simulink model "requirements"  (R2022a)
settings: Solver=FixedStepAuto  StartTime=0.0  StopTime=10.0  FixedStep=1e-3  RelTol=1e-3  EnableMultiTasking=on
settings Model: ExtModeTrigDuration=5  Creator=zaree  LastModifiedBy=zaree
settings OptimizationCC: EnhancedBackFolding=on  PassReuseOutputArgsAs=Individual arguments  ZeroExternalMemoryAtStartup=off  ZeroInternalMemoryAtStartup=off  MaxStackSize=64  OptimizeBlockOrder=speed  DifferentSizesBufferReuse=on  OptimizationCustomize=off  EfficientTunableParamExpr=on
settings DebuggingCC: ParameterTunabilityLossMsg=error
settings HardwareCC: ProdBitPerPointer=32  ProdBitPerSizeT=32  ProdBitPerPtrDiffT=32  ProdLargestAtomicInteger=Long  ProdLargestAtomicFloat=Double  ProdWordSize=32  ProdHWDeviceType=ARM Compatible->ARM Cortex
settings SFSimCC: MATLABDynamicMemAlloc=off
settings RTWCC: SystemTargetFile=ert.tlc  HardwareBoard=NXP FRDM-K64F  TLCOptions="-aInlineSetEventsForThisBaseRateFcn=TLC_FALSE -aSuppressMultiTaskScheduler=TLC_FALSE  -aRateBasedStepFcn=0"  TemplateMakefile=ert_default_tmf  Toolchain=GNU Tools for ARM Embedded Processors
settings CodeAppCC: ForceParamTrailComments=on  IgnoreCustomStorageClasses=off  OperatorAnnotations=on  SimulinkDataObjDesc=on  SFDataObjDesc=on  InsertBlockDesc=on
settings ERTTargetCC: ExtModeTransport=4  ExtModeMexFile=sendToCommService

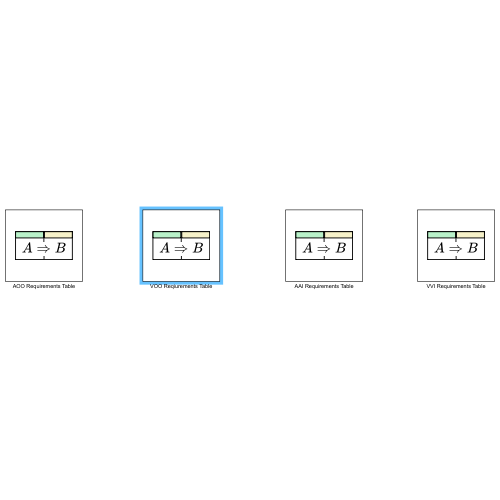
[thumbnail: Simulink's stored preview of the top-level diagram]
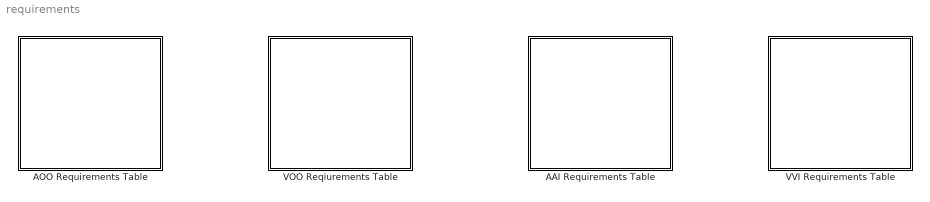
== system requirements ==
  AAI Requirements Table : Requirements Table  TreatAsAtomicUnit=on
  AOO Requirements Table : Requirements Table  TreatAsAtomicUnit=on
  VOO Reqiurements Table : Requirements Table  TreatAsAtomicUnit=on
  VVI Requirements Table : Requirements Table  TreatAsAtomicUnit=on

== stateflow chart requirements/VOO Reqiurements Table ==
  (default) -> (junction 1073741860)
  (junction 1073741860) -> (junction 1073741861) : {
      | % SF_REQ_REV_07
      | }
  (junction 1073741861) -> (junction 1073741863) : {
      | % HEADER_ASSIGNMENTS
      |
      | }
  (junction 1073741863) -> (junction 1073741865) : {
      | % START_A_4
      | }
  (junction 1073741865) -> (junction 1073741867) : {
      | }
  (junction 1073741867) -> (junction 1073741869)
  (junction 1073741869) -> (junction 1073741871) : {
      | }
  (junction 1073741871) -> (junction 1073741873) : {
      | % END_A_4
      | }
  (junction 1073741873) -> (junction 1073741898) : {
      | % START_R_1
      | }
  (junction 1073741898) -> (junction 1073741900) : {
      | }
  (junction 1073741900) -> (junction 1073741902) : {
      |
      |
      | }
  (junction 1073741902) -> (junction 1073741904) : {
      | }
  (junction 1073741904) -> (junction 1073741906) : {
      | % END_R_1
      | }
  (junction 1073741906) -> (junction 1073741910) : {
      | % START_R_7
      | }
  (junction 1073741910) -> (junction 1073741912) : {
      | }
  (junction 1073741912) -> (junction 1073741914) : {
      |
      |
      | }
  (junction 1073741914) -> (junction 1073741916) : {
      | }
  (junction 1073741916) -> (junction 1073741918) : {
      | % END_R_7
      | }

== stateflow chart requirements/VVI Requirements Table ==
  (default) -> (junction 1073741999)
  (junction 1073741999) -> (junction 1073742000) : {
      | % SF_REQ_REV_07
      | }
  (junction 1073742000) -> (junction 1073742002) : {
      | % HEADER_ASSIGNMENTS
      |
      | }
  (junction 1073742002) -> (junction 1073742004) : {
      | % START_A_4
      | }
  (junction 1073742004) -> (junction 1073742006) : {
      | }
  (junction 1073742006) -> (junction 1073742008)
  (junction 1073742008) -> (junction 1073742010) : {
      | }
  (junction 1073742010) -> (junction 1073742030) : {
      | % END_A_4
      | }
  (junction 1073742030) -> (junction 1073742066) : {
      | % START_R_10
      | }
  (junction 1073742066) -> (junction 1073742068) : {
      | }
  (junction 1073742068) -> (junction 1073742070) : {
      |
      |
      | }
  (junction 1073742070) -> (junction 1073742072) : {
      | }
  (junction 1073742072) -> (junction 1073742074) : {
      | % END_R_10
      | }
  (junction 1073742074) -> (junction 1073742078) : {
      | % START_R_1
      | }
  (junction 1073742078) -> (junction 1073742080) : {
      | }
  (junction 1073742080) -> (junction 1073742082)
  (junction 1073742082) -> (junction 1073742084) [order 1] : [duration((PACE_CHARGE_CTRL == 1) && (VENT_PACE_CTRL == 1) && (VENT_GND_CTRL == 0) && (PACE_GND_CTRL == 0 ) && (Z_VENT_CTRL == 0) && (VENT_CMP_DETECT ==1)) >= f_waitInterval]
  (junction 1073742082) -> (junction 1073742090) [order 2]
  (junction 1073742084) -> (junction 1073742086) : {
      | reqtable_postcondition((PACE_CHARGE_CTRL == 1) && (VENT_PACE_CTRL == 1) && (VENT_GND_CTRL == 0) && (PACE_GND_CTRL == 0) && (Z_VENT_CTRL == 0) && (VENT_CMP_DETECT ==1), 'R:2');
      | SENSE
      |
      | }
  (junction 1073742086) -> (junction 1073742088) : {
      | }
  (junction 1073742088) -> (junction 1073742090)
  (junction 1073742090) -> (junction 1073742092)
  (junction 1073742092) -> (junction 1073742094) : {
      | % END_R_1
      | }
  (junction 1073742094) -> (junction 1073742045) : {
      | % START_R_7
      | }
  (junction 1073742045) -> (junction 1073742047) : {
      | }
  (junction 1073742047) -> (junction 1073742049)
  (junction 1073742049) -> (junction 1073742051) [order 1] : [duration((PACE_CHARGE_CTRL == 1) && (VENT_PACE_CTRL == 1) && (VENT_GND_CTRL == 0) && (PACE_GND_CTRL == 0) && (Z_VENT_CTRL == 0) && (VENT_CMP_DETECT ==0)) >= f_waitInterval]
  (junction 1073742049) -> (junction 1073742057) [order 2]
  (junction 1073742051) -> (junction 1073742053) : {
      | reqtable_postcondition((PACE_CHARGE_CTRL == 0) && (VENT_PACE_CTRL == 1) && (VENT_GND_CTRL == 0) && (PACE_GND_CTRL == 1) && (Z_VENT_CTRL == 0) && (VENT_CMP_DETECT ==1), 'R:3');
      | PACE
      |
      | }
  (junction 1073742053) -> (junction 1073742055) : {
      | }
  (junction 1073742055) -> (junction 1073742057)
  (junction 1073742057) -> (junction 1073742059)
  (junction 1073742059) -> (junction 1073742061) : {
      | % END_R_7
      | }

== stateflow chart requirements/AOO Requirements Table ==
  (default) -> (junction 1073742591)
  (junction 1073742591) -> (junction 1073742592) : {
      | % SF_REQ_REV_07
      | }
  (junction 1073742592) -> (junction 1073742594) : {
      | % HEADER_ASSIGNMENTS
      |
      | }
  (junction 1073742594) -> (junction 1073742596) : {
      | % START_A_4
      | }
  (junction 1073742596) -> (junction 1073742598) : {
      | }
  (junction 1073742598) -> (junction 1073742600)
  (junction 1073742600) -> (junction 1073742602) : {
      | }
  (junction 1073742602) -> (junction 1073742604) : {
      | % END_A_4
      | }
  (junction 1073742604) -> (junction 1073742606) : {
      | % START_R_1
      | }
  (junction 1073742606) -> (junction 1073742608) : {
      | }
  (junction 1073742608) -> (junction 1073742610)
  (junction 1073742610) -> (junction 1073742612) [order 1] : [(PACE_CHARGE_CTRL == 0) && (ATR_CHARGE_CTRL == 1) && (ATR_GND_CTRL == 0) && (PACE_GND_CTRL == 1) && (Z_ATR_CTRL == 0)]
  (junction 1073742610) -> (junction 1073742618) [order 2]
  (junction 1073742612) -> (junction 1073742614) : {
      | reqtable_postcondition((PACE_CHARGE_CTRL == 1) && (ATR_PACE_CTRL == 0) && (ATR_GND_CTRL == 1) && (PACE_GND_CTRL == 1) && (Z_ATR_CTRL == 0), 'R:1');
      |
      |
      | }
  (junction 1073742614) -> (junction 1073742616) : {
      | }
  (junction 1073742616) -> (junction 1073742618)
  (junction 1073742618) -> (junction 1073742620)
  (junction 1073742620) -> (junction 1073742622) : {
      | % END_R_1
      | }
  (junction 1073742622) -> (junction 1073742624) : {
      | % START_R_7
      | }
  (junction 1073742624) -> (junction 1073742626) : {
      | }
  (junction 1073742626) -> (junction 1073742628)
  (junction 1073742628) -> (junction 1073742630) [order 1] : [(PACE_CHARGE_CTRL == 1) && (ATR_PACE_CTRL==0) && (ATR_GND_CTRL==1) && (PACE_GND_CTRL == 1) && (Z_ATR_CTRL == 0)]
  (junction 1073742628) -> (junction 1073742636) [order 2]
  (junction 1073742630) -> (junction 1073742632) : {
      | reqtable_postcondition((PACE_CHARGE_CTRL == 0) && (ATR_CHARGE_CTRL == 1) && (ATR_GND_CTRL == 0) && (PACE_GND_CTRL == 1) && (Z_ATR_CTRL == 0), 'R:2');
      |
      |
      | }
  (junction 1073742632) -> (junction 1073742634) : {
      | }
  (junction 1073742634) -> (junction 1073742636)
  (junction 1073742636) -> (junction 1073742638)
  (junction 1073742638) -> (junction 1073742640) : {
      | % END_R_7
      | }
  (junction 1073742640) -> (junction 1073742642) : {
      | % START_R_10
      | }
  (junction 1073742642) -> (junction 1073742644) : {
      | }
  (junction 1073742644) -> (junction 1073742646)
  (junction 1073742646) -> (junction 1073742648) [order 1] : [(PACE_CHARGE_CTRL == 0) && (VENT_PACE_CTRL == 1) && (VENT_GND_CTRL == 0) && (PACE_GND_CTRL == 1) && (Z_VENT_CTRL == 0)]
  (junction 1073742646) -> (junction 1073742654) [order 2]
  (junction 1073742648) -> (junction 1073742650) : {
      | reqtable_postcondition((PACE_CHARGE_CTRL == 1) && (VENT_CHARGE_CTRL == 0) && (VENT_GND_CTRL == 1) && (PACE_GND_CTRL == 1) && (Z_VENT_CTRL == 0), 'R:3');
      |
      |
      | }
  (junction 1073742650) -> (junction 1073742652) : {
      | }
  (junction 1073742652) -> (junction 1073742654)
  (junction 1073742654) -> (junction 1073742656)
  (junction 1073742656) -> (junction 1073742658) : {
      | % END_R_10
      | }
  (junction 1073742658) -> (junction 1073742660) : {
      | % START_R_13
      | }
  (junction 1073742660) -> (junction 1073742662) : {
      | }
  (junction 1073742662) -> (junction 1073742664)
  (junction 1073742664) -> (junction 1073742666) [order 1] : [(PACE_CHARGE_CTRL == 1) && (VENT_PACE_CTRL == 0) && (VENT_GND_CTRL == 1) && (PACE_GND_CTRL == 1) && (Z_VENT_CTRL == 0)]
  (junction 1073742664) -> (junction 1073742672) [order 2]
  (junction 1073742666) -> (junction 1073742668) : {
      | reqtable_postcondition((PACE_CHARGE_CTRL == 0) && (VENT_CHARGE_CTRL == 1) && (VENT_GND_CTRL == 0) && (PACE_GND_CTRL == 1) && (Z_VENT_CTRL == 0), 'R:4');
      |
      |
      | }
  (junction 1073742668) -> (junction 1073742670) : {
      | }
  (junction 1073742670) -> (junction 1073742672)
  (junction 1073742672) -> (junction 1073742674)
  (junction 1073742674) -> (junction 1073742676) : {
      | % END_R_13
      | }
  (junction 1073742676) -> (junction 1073742766) : {
      | % START_R_22
      | }
  (junction 1073742766) -> (junction 1073742768) : {
      | }
  (junction 1073742768) -> (junction 1073742770)
  (junction 1073742770) -> (junction 1073742772) [order 1] : [duration((PACE_CHARGE_CTRL == 1) && (ATR_PACE_CTRL == 1) && (ATR_GND_CTRL == 0) && (PACE_GND_CTRL == 0 ) && (Z_ATR_CTRL == 0) && (ATR_CMP_DETECT ==1)) >= VRP]
  (junction 1073742770) -> (junction 1073742778) [order 2]
  (junction 1073742772) -> (junction 1073742774) : {
      | reqtable_postcondition((PACE_CHARGE_CTRL == 1) && (ATR_PACE_CTRL == 1) && (ATR_GND_CTRL == 0) && (PACE_GND_CTRL == 0) && (Z_ATR_CTRL == 0) && (ATR_CMP_DETECT ==1), 'R:5');
      | SENSE
      |
      | }
  (junction 1073742774) -> (junction 1073742776) : {
      | }
  (junction 1073742776) -> (junction 1073742778)
  (junction 1073742778) -> (junction 1073742780)
  (junction 1073742780) -> (junction 1073742782) : {
      | % END_R_22
      | }
  (junction 1073742782) -> (junction 1073742787) : {
      | % START_R_25
      | }
  (junction 1073742787) -> (junction 1073742789) : {
      | }
  (junction 1073742789) -> (junction 1073742791)
  (junction 1073742791) -> (junction 1073742793) [order 1] : [duration((PACE_CHARGE_CTRL == 1) && (ATR_PACE_CTRL == 1) && (ATR_GND_CTRL == 0) && (PACE_GND_CTRL == 0) && (Z_ATR_CTRL == 0) && (ATR_CMP_DETECT ==0)) >= NOT_Atrium_Pulse_Width - VRP]
  (junction 1073742791) -> (junction 1073742799) [order 2]
  (junction 1073742793) -> (junction 1073742795) : {
      | reqtable_postcondition((PACE_CHARGE_CTRL == 0) && (ATR_PACE_CTRL == 1) && (ATR_GND_CTRL == 0) && (PACE_GND_CTRL == 1) && (Z_ATR_CTRL == 0) && (ATR_CMP_DETECT ==0), 'R:6');
      | PACE
      |
      | }
  (junction 1073742795) -> (junction 1073742797) : {
      | }
  (junction 1073742797) -> (junction 1073742799)
  (junction 1073742799) -> (junction 1073742801)
  (junction 1073742801) -> (junction 1073742803) : {
      | % END_R_25
      | }
  (junction 1073742803) -> (junction 1073742820) : {
      | % START_R_34
      | }
  (junction 1073742820) -> (junction 1073742822) : {
      | }
  (junction 1073742822) -> (junction 1073742824)
  (junction 1073742824) -> (junction 1073742826) [order 1] : [duration((PACE_CHARGE_CTRL == 0) && (ATR_PACE_CTRL == 1) && (ATR_GND_CTRL == 0) && (PACE_GND_CTRL == 1) && (Z_ATR_CTRL == 0) && (ATR_CMP_DETECT ==1)) >= Atrium_Pulse_Width]
  (junction 1073742824) -> (junction 1073742832) [order 2]
  (junction 1073742826) -> (junction 1073742828) : {
      | reqtable_postcondition((PACE_CHARGE_CTRL == 1) && (ATR_PACE_CTRL == 1) && (ATR_GND_CTRL == 0) && (PACE_GND_CTRL == 0 ) && (Z_ATR_CTRL == 0) && (ATR_CMP_DETECT ==1), 'R:7');
      | SENSE
      |
      | }
  (junction 1073742828) -> (junction 1073742830) : {
      | }
  (junction 1073742830) -> (junction 1073742832)
  (junction 1073742832) -> (junction 1073742834)
  (junction 1073742834) -> (junction 1073742836) : {
      | % END_R_34
      | }
  (junction 1073742836) -> (junction 1073742724) : {
      | % START_R_28
      | }
  (junction 1073742724) -> (junction 1073742726) : {
      | }
  (junction 1073742726) -> (junction 1073742728)
  (junction 1073742728) -> (junction 1073742730) [order 1] : [duration((PACE_CHARGE_CTRL == 1) && (VENT_PACE_CTRL == 1) && (VENT_GND_CTRL == 0) && (PACE_GND_CTRL == 0 ) && (Z_VENT_CTRL == 0) && (VENT_CMP_DETECT ==1)) >= VRP]
  (junction 1073742728) -> (junction 1073742736) [order 2]
  (junction 1073742730) -> (junction 1073742732) : {
      | reqtable_postcondition((PACE_CHARGE_CTRL == 1) && (VENT_PACE_CTRL == 1) && (VENT_GND_CTRL == 0) && (PACE_GND_CTRL == 0) && (Z_VENT_CTRL == 0) && (VENT_CMP_DETECT ==1), 'R:8');
      | SENSE
      |
      | }
  (junction 1073742732) -> (junction 1073742734) : {
      | }
  (junction 1073742734) -> (junction 1073742736)
  (junction 1073742736) -> (junction 1073742738)
  (junction 1073742738) -> (junction 1073742740) : {
      | % END_R_28
      | }
  (junction 1073742740) -> (junction 1073742745) : {
      | % START_R_31
      | }
  (junction 1073742745) -> (junction 1073742747) : {
      | }
  (junction 1073742747) -> (junction 1073742749)
  (junction 1073742749) -> (junction 1073742751) [order 1] : [duration((PACE_CHARGE_CTRL == 1) && (VENT_PACE_CTRL == 1) && (VENT_GND_CTRL == 0) && (PACE_GND_CTRL == 0) && (Z_VENT_CTRL == 0) && (VENT_CMP_DETECT ==0)) >= NOT_Ventricular_Pulse_Width - VRP]
  (junction 1073742749) -> (junction 1073742757) [order 2]
  (junction 1073742751) -> (junction 1073742753) : {
      | reqtable_postcondition((PACE_CHARGE_CTRL == 0) && (VENT_PACE_CTRL == 1) && (VENT_GND_CTRL == 0) && (PACE_GND_CTRL == 1) && (Z_VENT_CTRL == 0) && (VENT_CMP_DETECT ==0), 'R:9');
      | PACE
      |
      | }
  (junction 1073742753) -> (junction 1073742755) : {
      | }
  (junction 1073742755) -> (junction 1073742757)
  (junction 1073742757) -> (junction 1073742759)
  (junction 1073742759) -> (junction 1073742761) : {
      | % END_R_31
      | }
  (junction 1073742761) -> (junction 1073742853) : {
      | % START_R_37
      | }
  (junction 1073742853) -> (junction 1073742855) : {
      | }
  (junction 1073742855) -> (junction 1073742857)
  (junction 1073742857) -> (junction 1073742859) [order 1] : [duration((PACE_CHARGE_CTRL == 0) && (VENT_PACE_CTRL == 1) && (VENT_GND_CTRL == 0) && (PACE_GND_CTRL == 1) && (Z_VENT_CTRL == 0) && (VENT_CMP_DETECT ==0)) >= Ventricular_Pulse_Width]
  (junction 1073742857) -> (junction 1073742865) [order 2]
  (junction 1073742859) -> (junction 1073742861) : {
      | reqtable_postcondition((PACE_CHARGE_CTRL == 1) && (VENT_PACE_CTRL == 1) && (VENT_GND_CTRL == 0) && (PACE_GND_CTRL == 0 ) && (Z_VENT_CTRL == 0) && (VENT_CMP_DETECT ==1), 'R:10');
      | SENSE
      |
      | }
  (junction 1073742861) -> (junction 1073742863) : {
      | }
  (junction 1073742863) -> (junction 1073742865)
  (junction 1073742865) -> (junction 1073742867)
  (junction 1073742867) -> (junction 1073742869) : {
      | % END_R_37
      | }

== stateflow chart requirements/AAI Requirements Table ==
  (default) -> (junction 1073741963)
  (junction 1073741963) -> (junction 1073741964) : {
      | % SF_REQ_REV_07
      | }
  (junction 1073741964) -> (junction 1073741966) : {
      | % HEADER_ASSIGNMENTS
      |
      | }
  (junction 1073741966) -> (junction 1073741968) : {
      | % START_A_4
      | }
  (junction 1073741968) -> (junction 1073741970) : {
      | }
  (junction 1073741970) -> (junction 1073741972)
  (junction 1073741972) -> (junction 1073741974) : {
      | }
  (junction 1073741974) -> (junction 1073741976) : {
      | % END_A_4
      | }
  (junction 1073741976) -> (junction 1073741978) : {
      | % START_R_1
      | }
  (junction 1073741978) -> (junction 1073741980) : {
      | }
  (junction 1073741980) -> (junction 1073741982)
  (junction 1073741982) -> (junction 1073741984) [order 1] : [duration((PACE_CHARGE_CTRL == 1) && (ATR_PACE_CTRL == 1) && (ATR_GND_CTRL == 0) && (PACE_GND_CTRL == 0 ) && (Z_ATR_CTRL == 0) && (ATR_CMP_DETECT ==1)) >= f_waitInterval]
  (junction 1073741982) -> (junction 1073741990) [order 2]
  (junction 1073741984) -> (junction 1073741986) : {
      | reqtable_postcondition((PACE_CHARGE_CTRL == 1) && (ATR_PACE_CTRL == 1) && (ATR_GND_CTRL == 0) && (PACE_GND_CTRL == 0) && (Z_ATR_CTRL == 0) && (ATR_CMP_DETECT ==1), 'R:1');
      | SENSE
      |
      | }
  (junction 1073741986) -> (junction 1073741988) : {
      | }
  (junction 1073741988) -> (junction 1073741990)
  (junction 1073741990) -> (junction 1073741992)
  (junction 1073741992) -> (junction 1073741994) : {
      | % END_R_1
      | }
  (junction 1073741994) -> (junction 1073741996) : {
      | % START_R_7
      | }
  (junction 1073741996) -> (junction 1073741998) : {
      | }
  (junction 1073741998) -> (junction 1073742000)
  (junction 1073742000) -> (junction 1073742002) [order 1] : [duration((PACE_CHARGE_CTRL == 1) && (ATR_PACE_CTRL == 1) && (ATR_GND_CTRL == 0) && (PACE_GND_CTRL == 0) && (Z_ATR_CTRL == 0) && (ATR_CMP_DETECT ==0)) >= f_waitInterval]
  (junction 1073742000) -> (junction 1073742008) [order 2]
  (junction 1073742002) -> (junction 1073742004) : {
      | reqtable_postcondition((PACE_CHARGE_CTRL == 0) && (ATR_PACE_CTRL == 1) && (ATR_GND_CTRL == 0) && (PACE_GND_CTRL == 1) && (Z_ATR_CTRL == 0) && (ATR_CMP_DETECT ==1), 'R:2');
      | PACE
      |
      | }
  (junction 1073742004) -> (junction 1073742006) : {
      | }
  (junction 1073742006) -> (junction 1073742008)
  (junction 1073742008) -> (junction 1073742010)
  (junction 1073742010) -> (junction 1073742012) : {
      | % END_R_7
      | }
